simulink model "Simplus_Dual_Automated"  (R2022b)
settings: Solver=ode3  StartTime=0.0  StopTime=35  FixedStep=Ts  RelTol=1e-3  EnableMultiTasking=on
InitFcn:
  | Ts = 100e-6;
model workspace (MAT data in the model file):
  Fbase = 50
  Filter_Ind = 0.00435
  Shunt_C = 2.2e-06
  Test_Interval = 5
  Ts = 0.0001
  VDCref = 48
undefined symbols (not defined in the file): DiscIntNeverNeededParam
libraries: rtpi x45, spsabctodq0Lib x4, spsdq0toabcLib x2, simulink x1
(part 1 of 2)
settings Model: ModifiedByFormat=The MathWorks Inc.  SimulationMode=external  ExtModeTrigDuration=350000  ExtModeLogAll=off  Creator=The MathWorks, Inc.  LastModifiedBy=The MathWorks Inc.
settings SolverCC: AlgebraicLoopSolver=TrustRegion  PositivePriorityOrder=on  AutoInsertRateTranBlk=on
settings DataIOCC: LimitDataPoints=on  SaveFormat=Array  ReturnWorkspaceOutputs=off
settings OptimizationCC: EnhancedBackFolding=on  PassReuseOutputArgsThreshold=0  LocalBlockOutputs=off  EfficientMapNaN2IntZero=off  MaxStackSize=64  OptimizeBlockOrder=speed  DifferentSizesBufferReuse=on
settings DebuggingCC: UnderspecifiedInitializationDetection=Classic  MergeDetectMultiDrivingBlocksExec=none  SolverPrmCheckMsg=warning  ParameterTunabilityLossMsg=error  UnconnectedInputMsg=warning  UnconnectedOutputMsg=warning  UnconnectedLineMsg=warning  AllowSymbolicDim=off  SFUnexpectedBacktrackingDiag=warning  SFNoUnconditionalDefaultTransitionDiag=warning  SFExecutionAtInitializationDiag=none  SFMachineParentedDataDiag=warning  ArithmeticOperatorsInVariantConditions=warning
settings HardwareCC: ProdBitPerPointer=32  ProdBitPerSizeT=32  ProdBitPerPtrDiffT=32  ProdLargestAtomicInteger=Long  ProdLargestAtomicFloat=Double  ProdWordSize=32  ProdHWDeviceType=ARM Compatible->ARM Cortex  UseEmbeddedCoderFeatures=off
settings ModelReferenceCC: EnableRefExpFcnMdlSchedulingChecks=on  PropagateSignalLabelsOutOfModel=off
settings SFSimCC: SimUseLocalCustomCode=off  SimParseCustomCode=off  MATLABDynamicMemAlloc=off  CustomCodeUndefinedFunction=UseInterfaceOnly
settings RTWCC: Description=Simplus  SystemTargetFile=simplus.tlc  TemplateMakefile=simplex.tmf  RTWUseLocalCustomCode=off  RTWUseSimCustomCode=on  Toolchain=Simplus Xenomai ARM32  BuildConfiguration=Faster Runs
settings CodeAppCC: OperatorAnnotations=on  MangleLength=10  StateflowObjectComments=on
settings STFCustomTargetCC: TargetLangStandard=C99 (ISO)  GenerateFullHeader=off  ConcurrentExecutionCompliant=on  GRTInterface=on  UseToolchainInfoCompliant=on  SystemTargetFile=simplus.tlc
settings GRTTargetCC: GenerateFullHeader=off  ParMdlRefBuildCompliant=off  CompOptLevelCompliant=off  CombineOutputUpdateFcns=off  MatFileLogging=off  CPPClassGenCompliant=off  GRTInterface=on  ExtMode=on  ExtModeMexArgs='192.168.10.109', 0, 17725
settings ConfigComp: CovMetricSettings=dw  CovSaveCumulativeToWorkspaceVar=on  CovSaveSingleToWorkspaceVar=on  CovExternalEMLEnable=off  CovSFcnEnable=off

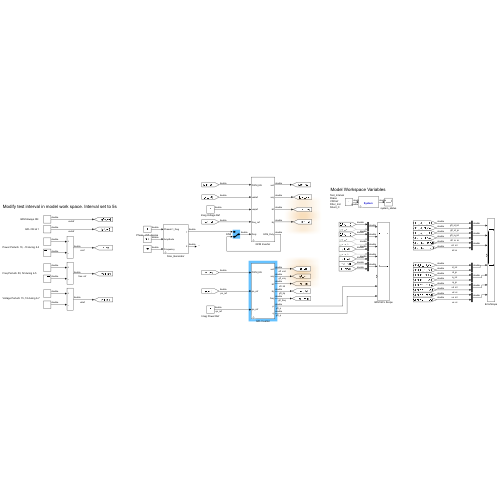
[thumbnail: Simulink's stored preview of the top-level diagram]
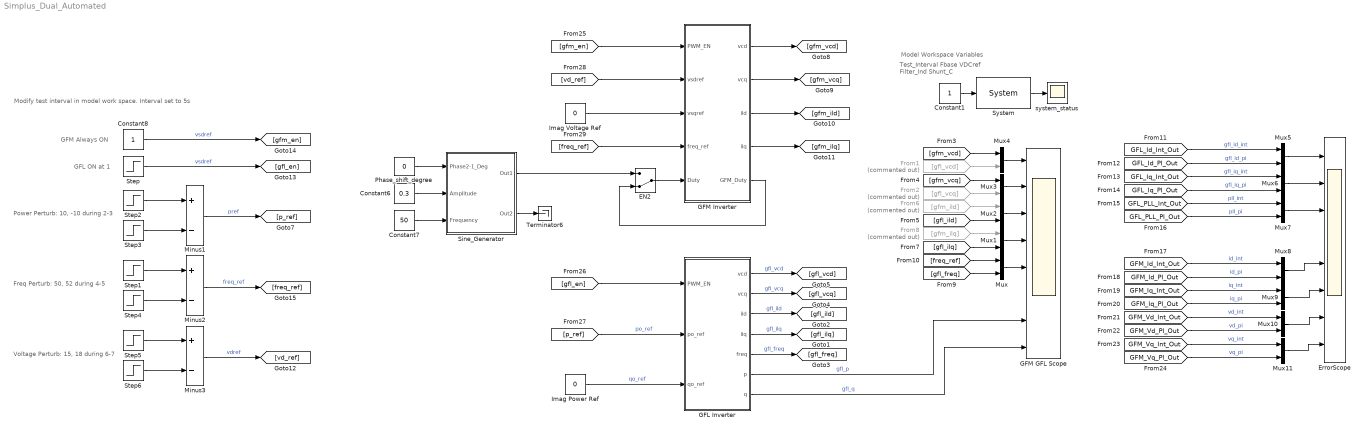
== system Simplus_Dual_Automated ==
  note: Test_Interval
      | Fbase
      | VDCref
      | Filter_Ind
      | Shunt_C
  note: Model Workspace Variables
  note: Modify test interval in model work space. Interval set to 5s
  note: GFM Always ON
  note: Power Perturb: 10, -10 during 2-3
  note: GFL ON at 1
  note: Freq Perturb: 50, 52 during 4-5
  note: Voltage Perturb: 15, 18 during 6-7
  Constant1 : Constant
  Constant6 : Constant  Value=0.3
  Constant7 : Constant  Value=50
  Constant8 : Constant
  EN2 : ManualSwitch  CurrentSetting=0
  ErrorScope : Scope  NumInputPorts=8
  From1 : From  Commented=on  GotoTag=gfl_vcd
      settings: CloseFcn=tagdialog Close
  From2 : From  Commented=on  GotoTag=gfl_vcq
      settings: CloseFcn=tagdialog Close
  From6 : From  Commented=on  GotoTag=gfm_ild
      settings: CloseFcn=tagdialog Close
  From8 : From  Commented=on  GotoTag=gfm_ilq
      settings: CloseFcn=tagdialog Close
  GFL Inverter : Subsystem  mask{Kp_PLL=6.09, Ki_PLL=9.57, IntSat_PLL=10000, Fcutoff=100, Id_Proportional=1.22, Id_Integral=957/16, I_SatLimit=200000}
      mask prompts: Kp_PLL "Proportional (P)"; Ki_PLL "Integral (I)"; IntSat_PLL "Saturator (Offset from 2*pi*Fbase)"; Fcutoff "LPF Cutoff Frequency (Hz)"; Id_Proportional "Proportional (P)"; Id_Integral "Integral (I)"; I_SatLimit "Integrator Saturation"
      mask DialogControl DescGroupVar Prompt: GFL Control Panel
      mask DialogControl DescTextVar Prompt: Modify current controller and PLL gains.
      mask DialogControl ParameterGroupVar_copy Prompt: PLL Parameters
      mask DialogControl Control2 Prompt: LPF is a first order LPF in the form  1/(2pi*f_c s + 1)
      mask DialogControl ParameterGroupVar Prompt: Current Controller Parameters
  GFM GFL Scope : Scope  NumInputPorts=8
  GFM Inverter : Subsystem  mask{Vd_Proportional=0.028, Vd_Integral=8.685*8, V_IntSat=1000, Id_Proportional=0.61, Id_Integral=240/16, I_IntSat=200000}
      mask prompts: Vd_Proportional "Proportional (P)"; Vd_Integral "Integral (I)"; V_IntSat "Integrator Saturator Limit"; Id_Proportional "Proportional (P)"; Id_Integral "Integral (I)"; I_IntSat "Integrator Saturator Limit"
      mask DialogControl DescGroupVar Prompt: GFM Control Panel
      mask DialogControl DescTextVar Prompt: Adjust gains and output/integrator limits for GFM voltage and current controllers
      mask DialogControl ParameterGroupVar_copy Prompt: Voltage Controller
      mask DialogControl ParameterGroupVar Prompt: Current Controller
  Imag Power Ref : Constant  Value=0
  Imag Voltage Ref : Constant  Value=0
  Minus1 : Sum  Inputs=+-
  Minus2 : Sum  Inputs=+-
  Minus3 : Sum  Inputs=+-
  Mux{,1..11} (12 alike) : Mux  Inputs=2
  Phase_shift_degree : Constant  Value=0
  Sine_Generator : Subsystem
  Step : Step  Time=Test_Interval*1
  Step1 : Step  Time=Test_Interval*4  Before=50  After=52
  Step2 : Step  Time=Test_Interval*2  Before=10  After=-10
  Step3 : Step  Time=Test_Interval*3  After=-20
  Step4 : Step  Time=Test_Interval*5  After=2
  Step5 : Step  Time=Test_Interval*6  Before=15  After=18
  Step6 : Step  Time=Test_Interval*7  After=3
  System : rtpi/System  Priority=-100  finger_print=015482637925  sync=Synchronous Series  div=4  estop=NONE
      settings: SourceProductName=Simplus Real-Time
  Terminator6 : Terminator
  system_status : Scope
  wires:
  System/1 -> system_status/1
  Constant1/1 -> System/1
  [gfm_en] -> GFM Inverter/1(PWM_EN)
  [vd_ref] -> GFM Inverter/2(vsdref)
  Imag Voltage Ref/1 -> GFM Inverter/3(vsqref)
  GFM Inverter/1(vcd) -> [gfm_vcd]
  GFM Inverter/2(vcq) -> [gfm_vcq]
  GFM Inverter/3(ild) -> [gfm_ild]
  GFM Inverter/4(ilq) -> [gfm_ilq]
  Mux3/1 -> GFM GFL Scope/2
  Mux4/1 -> GFM GFL Scope/1
  Mux2/1 -> GFM GFL Scope/3
  Mux1/1 -> GFM GFL Scope/4
  Mux/1 -> GFM GFL Scope/5
  [gfl_freq] -> Mux/2
  [freq_ref] -> Mux/1
  [gfl_ilq] -> Mux1/2
  From8/1 -> Mux1/1
  [gfl_ild] -> Mux2/2
  From6/1 -> Mux2/1
  From2/1 -> Mux3/2
  [gfm_vcq] -> Mux3/1
  From1/1 -> Mux4/2
  [gfm_vcd] -> Mux4/1
  Sine_Generator/1(Out1) -> EN2/1
  Constant6/1 -> Sine_Generator/2(Amplitude)
  Constant7/1 -> Sine_Generator/3(Frequency)
  Sine_Generator/2(Out2) -> Terminator6/1
  Phase_shift_degree/1 -> Sine_Generator/1(Phase2-1_Deg)
  GFM Inverter/5(GFM_Duty) -> EN2/2
  EN2/1 -> GFM Inverter/5(Duty)
  [gfl_en] -> GFL Inverter/1(PWM_EN)
  Imag Power Ref/1 -> GFL Inverter/3(qo_ref)  "qo_ref"
  GFL Inverter/2(vcq) -> [gfl_vcq]  "gfl_vcq"
  GFL Inverter/5(freq) -> [gfl_freq]  "gfl_freq"
  [p_ref] -> GFL Inverter/2(po_ref)  "po_ref"
  GFL Inverter/4(ilq) -> [gfl_ilq]  "gfl_ilq"
  GFL Inverter/6(p) -> GFM GFL Scope/7  "gfl_p"
  GFL Inverter/3(ild) -> [gfl_ild]  "gfl_ild"
  GFL Inverter/1(vcd) -> [gfl_vcd]  "gfl_vcd"
  GFL Inverter/7(q) -> GFM GFL Scope/8  "gfl_q"
  [GFL_Id_PI_Out] -> Mux5/2  "gfl_id_pi"
  Mux5/1 -> ErrorScope/1
  [GFL_Id_Int_Out] -> Mux5/1  "gfl_id_int"
  [GFL_Iq_Int_Out] -> Mux6/1  "gfl_iq_int"
  [GFL_Iq_PI_Out] -> Mux6/2  "gfl_iq_pi"
  Mux6/1 -> ErrorScope/2
  [GFL_PLL_Int_Out] -> Mux7/1  "pll_int"
  Mux7/1 -> ErrorScope/3
  [GFL_PLL_PI_Out] -> Mux7/2  "pll_pi"
  [GFM_Id_Int_Out] -> Mux8/1  "id_int"
  [GFM_Id_PI_Out] -> Mux8/2  "id_pi"
  Mux10/1 -> ErrorScope/7
  Mux8/1 -> ErrorScope/5
  [GFM_Vd_Int_Out] -> Mux10/1  "vd_int"
  [GFM_Iq_Int_Out] -> Mux9/1  "iq_int"
  Mux9/1 -> ErrorScope/6
  [GFM_Iq_PI_Out] -> Mux9/2  "iq_pi"
  [GFM_Vd_PI_Out] -> Mux10/2  "vd_pi"
  Mux11/1 -> ErrorScope/8
  [GFM_Vq_Int_Out] -> Mux11/1  "vq_int"
  [GFM_Vq_PI_Out] -> Mux11/2  "vq_pi"
  Step2/1 -> Minus1/1
  Step3/1 -> Minus1/2
  Step/1 -> [gfl_en]  "vsdref"
  Minus1/1 -> [p_ref]  "pref"
  Constant8/1 -> [gfm_en]  "vsdref"
  Minus2/1 -> [freq_ref]  "freq_ref"
  Step4/1 -> Minus2/2
  Step1/1 -> Minus2/1
  [freq_ref] -> GFM Inverter/4(freq_ref)
  Minus3/1 -> [vd_ref]  "vdref"
  Step6/1 -> Minus3/2
  Step5/1 -> Minus3/1

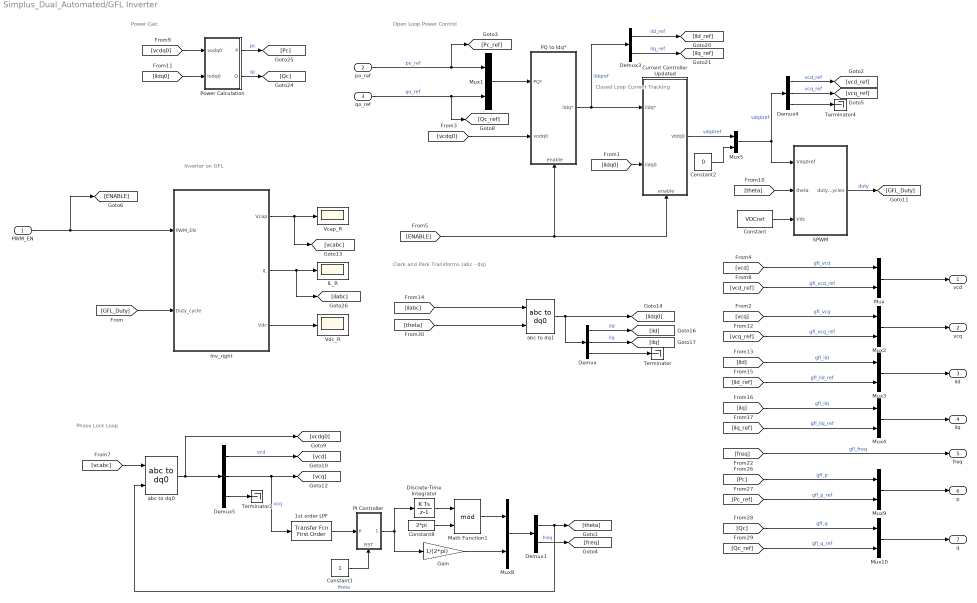
== system Simplus_Dual_Automated/GFL Inverter ==
  note: Clark and Park Transforms (abc - dq)
  note: Closed Loop Current Tracking
  note: Phase Lock Loop
  note: Inverter on GFL
  note: Power Calc
  note: Open Loop Power Control
  PWM_EN : Inport
  po_ref : Inport  Port=2
  qo_ref : Inport  Port=3
  1st order LPF : simulink/Discrete/Transfer Fcn First Order  PoleZ=exp(-2*pi*Fcutoff*Ts)  ICPrevOutput=0.0  DoSatur=off
  Constant : Constant  Value=VDCref
  Constant1 : Constant
  Constant2 : Constant  Value=0
  Constant8 : Constant  Value=2*pi
  Current Controller Updated : Subsystem
      settings: PortSchema="{\"entries\":[{\"content\":{\"sides\":[{\"content\":{\"connectorIds\":[\"In1\",\"In2\"]},\"type\":\"ConnectorPlacement.EquallySpacedRectSide\",\"uuid\":\"134caf41-c34b-48d0-a71a-522329c40d8c\"},{\"content\":{\"connectorIds\":[\"Out1\"],\"side\":\"RIGHT\"},\"type\":\"ConnectorPlacement.EquallySpacedRectSide\",\"uuid\":\"de6d8359-09d9-4cb7-8990-bc4b6d48f18d\"},{\"content\":{\"connectorIds\":[],\"side\":\"TOP\"},\"type\":\"ConnectorPlacement.EquallySpacedRectSide\",\"uuid\":\"e2785d07-2ead-4d42-94ac-8025f550e46a\"},{\"content\":{\"connectorIds\":[\"In3\"],\"side\":\"BOTTOM\"},\"type\":\"ConnectorPlacement.EquallySpacedRectSide\",\"uuid\":\"a912a274-012c-4cba-911c-beb79bb7dc91\"}]},\"type\":\"ConnectorPlacement.EquallySpacedConnector\",\"uuid\":\"3c498838-bb9a-4b09-bf48-00f71cabf7b4\"}],\"packageUris\":[\"http://schema.mathworks.com/mf0/Connector/R2020b\"],\"version\":\"1.0\"}"
  Demux : Demux  Outputs=3
  Demux1 : Demux  Outputs=2
  Demux3 : Demux  Outputs=2
  Demux4 : Demux  Outputs=3
  Demux5 : Demux  Outputs=3
  Discrete-Time Integrator : DiscreteIntegrator  SampleTime=Ts  ICPrevOutput=DiscIntNeverNeededParam  ICPrevScaledInput=DiscIntNeverNeededParam
  Gain : Gain  Gain=1/(2*pi)
  IL_R : Scope
  Inv_right : Subsystem
  Math Function1 : Math  Operator=mod  SignedPower=on
  Mux{,1..5,8..10} (9 alike) : Mux  Inputs=2
  PI Controller : Subsystem
      settings: PortSchema="{\"entries\":[{\"content\":{\"sides\":[{\"content\":{\"connectorIds\":[\"In1\"]},\"type\":\"ConnectorPlacement.EquallySpacedRectSide\",\"uuid\":\"de74edf3-48e0-492f-8bd8-cb8fa34f4920\"},{\"content\":{\"connectorIds\":[\"Out1\"],\"side\":\"RIGHT\"},\"type\":\"ConnectorPlacement.EquallySpacedRectSide\",\"uuid\":\"732ba37e-c2f5-4a41-96c7-cf5d66f1810a\"},{\"content\":{\"connectorIds\":[],\"side\":\"TOP\"},\"type\":\"ConnectorPlacement.EquallySpacedRectSide\",\"uuid\":\"cc9767f0-3de2-493b-9176-a3d2c83c4b10\"},{\"content\":{\"connectorIds\":[\"In2\"],\"side\":\"BOTTOM\"},\"type\":\"ConnectorPlacement.EquallySpacedRectSide\",\"uuid\":\"a440190f-f792-4428-a915-fb5e20f94e16\"}]},\"type\":\"ConnectorPlacement.EquallySpacedConnector\",\"uuid\":\"ab91a7bc-5a4b-4de4-8ccc-ccc371bac732\"}],\"packageUris\":[\"http://schema.mathworks.com/mf0/Connector/R2020b\"],\"version\":\"1.0\"}"
  PQ to Idq* : Subsystem
      settings: PortSchema="{\"entries\":[{\"content\":{\"sides\":[{\"content\":{\"connectorIds\":[\"In1\",\"In2\"]},\"type\":\"ConnectorPlacement.EquallySpacedRectSide\",\"uuid\":\"5271b3ed-46a4-4113-9b69-458d23b85fa2\"},{\"content\":{\"connectorIds\":[\"Out1\"],\"side\":\"RIGHT\"},\"type\":\"ConnectorPlacement.EquallySpacedRectSide\",\"uuid\":\"00fb532b-4b50-4607-a5c4-cd74a5a5fc42\"},{\"content\":{\"connectorIds\":[],\"side\":\"TOP\"},\"type\":\"ConnectorPlacement.EquallySpacedRectSide\",\"uuid\":\"05671b8e-b1fa-45d3-a4a8-1640aa1af326\"},{\"content\":{\"connectorIds\":[\"In3\"],\"side\":\"BOTTOM\"},\"type\":\"ConnectorPlacement.EquallySpacedRectSide\",\"uuid\":\"cfa1ca65-6f63-4245-906b-c8bf76b96ed3\"}]},\"type\":\"ConnectorPlacement.EquallySpacedConnector\",\"uuid\":\"bf062c94-390f-4409-83d1-f8a32d59f496\"}],\"packageUris\":[\"http://schema.mathworks.com/mf0/Connector/R2020b\"],\"version\":\"1.0\"}"
  Power Calculation : Subsystem
  SPWM : Subsystem
  Terminator : Terminator
  Terminator2 : Terminator
  Terminator4 : Terminator
  Vcap_R : Scope
  Vdc_R : Scope
  abc to dq0 : spsabctodq0Lib/abc to dq0  Alignment=90 degrees behind phase A axis
  abc to dq1 : spsabctodq0Lib/abc to dq0  Alignment=90 degrees behind phase A axis
  vcd : Outport
  vcq : Outport  Port=2
  ild : Outport  Port=3
  ilq : Outport  Port=4
  freq : Outport  Port=5
  p : Outport  Port=6
  q : Outport  Port=7
  wires:
  [ild] -> Mux3/1  "gfl_ild"
  Demux1/1 -> abc to dq0/2, [theta]  "theta"
  Inv_right/2(IL) -> [ilabc], IL_R/1
  Inv_right/1(Vcap) -> [vcabc], Vcap_R/1
  Mux5/1 -> Demux4/1, SPWM/1(Vdq0ref)  "vdq0ref"
  Demux3/1 -> [ild_ref]  "ild_ref"
  Demux5/2 -> 1st order LPF/1, [vcq]  "vcq"
  Math Function1/1 -> Mux8/1
  [ild_ref] -> Mux3/2  "gfl_ild_ref"
  Power Calculation/1(P) -> [Pc]  "pc"
  [Pc_ref] -> Mux9/2  "gfl_p_ref"
  Power Calculation/2(Q) -> [Qc]  "qc"
  [vcabc] -> abc to dq0/1
  Constant/1 -> SPWM/3(Vdc)
  Demux/2 -> [ilq]  "ilq"
  Demux3/2 -> [ilq_ref]  "ilq_ref"
  [theta] -> SPWM/2(theta)
  Demux/3 -> Terminator/1
  [Qc] -> Mux10/1  "gfl_q"
  SPWM/1(duty_cycles) -> [GFL_Duty]  "duty"
  abc to dq0/1 -> [vcdq0], Demux5/1
  qo_ref/1 -> [Qc_ref], Mux1/2  "qo_ref"
  Demux4/2 -> [vcq_ref]  "vcq_ref"
  [ilq_ref] -> Mux4/2  "gfl_ilq_ref"
  Demux/1 -> [ild]  "ild"
  PQ to Idq*/1(iIdq*) -> Current Controller Updated/1(ildq*), Demux3/1  "ildqref"
  Demux4/3 -> Terminator4/1
  [vcq_ref] -> Mux2/2  "gfl_vcq_ref"
  [vcdq0] -> Power Calculation/1(vodq0)
  Discrete-Time Integrator/1 -> Math Function1/1
  PWM_EN/1 -> Inv_right/1(PWM_EN), [ENABLE]
  [theta] -> abc to dq1/2
  Gain/1 -> Mux8/2
  [vcd] -> Mux/1  "gfl_vcd"
  Mux1/1 -> PQ to Idq*/1(PQ*)
  Constant8/1 -> Math Function1/2
  [vcd_ref] -> Mux/2  "gfl_vcd_ref"
  Demux1/2 -> [freq]  "freq"
  [vcq] -> Mux2/1  "gfl_vcq"
  abc to dq1/1 -> [ildq0], Demux/1
  [ilq] -> Mux4/1  "gfl_ilq"
  Mux8/1 -> Demux1/1
  [ildq0] -> Current Controller Updated/2(ildq0)
  [Pc] -> Mux9/1  "gfl_p"
  Demux5/1 -> [vcd]  "vcd"
  [vcdq0] -> PQ to Idq*/2(vodq0)
  Demux5/3 -> Terminator2/1
  Inv_right/3(Vdc) -> Vdc_R/1
  [ildq0] -> Power Calculation/2(iodq0)
  [Qc_ref] -> Mux10/2  "gfl_q_ref"
  [ilabc] -> abc to dq1/1
  [GFL_Duty] -> Inv_right/2(Duty_cycle)
  po_ref/1 -> [Pc_ref], Mux1/1  "po_ref"
  Demux4/1 -> [vcd_ref]  "vcd_ref"
  PI Controller/1(Out) -> Gain/1, Discrete-Time Integrator/1
  Mux4/1 -> ilq/1
  Mux/1 -> vcd/1
  Mux3/1 -> ild/1
  Mux9/1 -> p/1
  Mux10/1 -> q/1
  Mux2/1 -> vcq/1
  [freq] -> freq/1  "gfl_freq"
  [ENABLE] -> Current Controller Updated/3(enable), PQ to Idq*/3(enable)
  Current Controller Updated/1(vtdq0) -> Mux5/1  "vdq0ref"
  Constant2/1 -> Mux5/2
  1st order LPF/1 -> PI Controller/1(e)
  Constant1/1 -> PI Controller/2(RST)

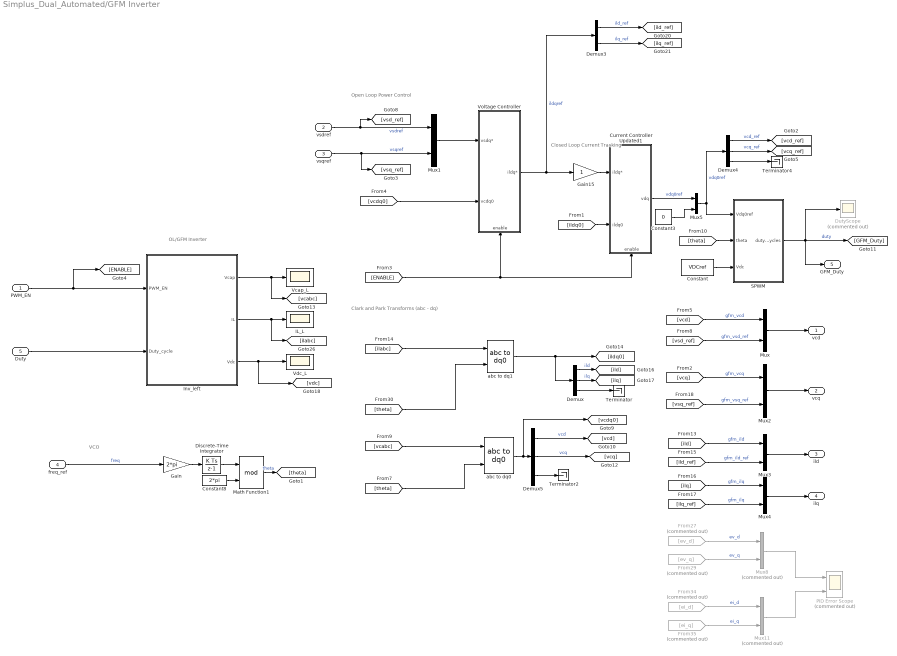
== system Simplus_Dual_Automated/GFM Inverter ==
  note: OL/GFM Inverter
  note: Open Loop Power Control
  note: VCO
  note: Clark and Park Transforms (abc - dq)
  note: Closed Loop Current Tracking
  PWM_EN : Inport
  vsdref : Inport  Port=2
  vsqref : Inport  Port=3
  freq_ref : Inport  Port=4
  Duty : Inport  Port=5
  Constant : Constant  Value=VDCref
  Constant3 : Constant  Value=0
  Constant8 : Constant  Value=2*pi
  Current Controller Updated1 : Subsystem
      settings: PortSchema="{\"entries\":[{\"content\":{\"sides\":[{\"content\":{\"connectorIds\":[\"In1\",\"In2\"]},\"type\":\"ConnectorPlacement.EquallySpacedRectSide\",\"uuid\":\"134caf41-c34b-48d0-a71a-522329c40d8c\"},{\"content\":{\"connectorIds\":[\"Out1\"],\"side\":\"RIGHT\"},\"type\":\"ConnectorPlacement.EquallySpacedRectSide\",\"uuid\":\"de6d8359-09d9-4cb7-8990-bc4b6d48f18d\"},{\"content\":{\"connectorIds\":[],\"side\":\"TOP\"},\"type\":\"ConnectorPlacement.EquallySpacedRectSide\",\"uuid\":\"e2785d07-2ead-4d42-94ac-8025f550e46a\"},{\"content\":{\"connectorIds\":[\"In3\"],\"side\":\"BOTTOM\"},\"type\":\"ConnectorPlacement.EquallySpacedRectSide\",\"uuid\":\"a912a274-012c-4cba-911c-beb79bb7dc91\"}]},\"type\":\"ConnectorPlacement.EquallySpacedConnector\",\"uuid\":\"3c498838-bb9a-4b09-bf48-00f71cabf7b4\"}],\"packageUris\":[\"http://schema.mathworks.com/mf0/Connector/R2020b\"],\"version\":\"1.0\"}"
  Demux : Demux  Outputs=3
  Demux3 : Demux  Outputs=2
  Demux4 : Demux  Outputs=3
  Demux5 : Demux  Outputs=3
  Discrete-Time Integrator : DiscreteIntegrator  SampleTime=Ts  ICPrevOutput=DiscIntNeverNeededParam  ICPrevScaledInput=DiscIntNeverNeededParam
  DutyScope : Scope  Commented=on
  From27 : From  Commented=on  GotoTag=ev_d
      settings: CloseFcn=tagdialog Close
  From29 : From  Commented=on  GotoTag=ev_q
      settings: CloseFcn=tagdialog Close
  From34 : From  Commented=on  GotoTag=ei_d
      settings: CloseFcn=tagdialog Close
  From35 : From  Commented=on  GotoTag=ei_q
      settings: CloseFcn=tagdialog Close
  Gain : Gain  Gain=2*pi
  Gain15 : Gain
  IL_L : Scope
  Inv_left : Subsystem
  Math Function1 : Math  Operator=mod  SignedPower=on
  Mux{,1..5} (6 alike) : Mux  Inputs=2
  Mux11 : Mux  Commented=on  Inputs=2
  Mux8 : Mux  Commented=on  Inputs=2
  PID Error Scope : Scope  Commented=on  NumInputPorts=2
  SPWM : Subsystem
  Terminator : Terminator
  Terminator2 : Terminator
  Terminator4 : Terminator
  Vcap_L : Scope
  Vdc_L : Scope
  Voltage Controller : Subsystem
      settings: PortSchema="{\"entries\":[{\"content\":{\"sides\":[{\"content\":{\"connectorIds\":[\"In1\",\"In2\"]},\"type\":\"ConnectorPlacement.EquallySpacedRectSide\",\"uuid\":\"134caf41-c34b-48d0-a71a-522329c40d8c\"},{\"content\":{\"connectorIds\":[\"Out1\"],\"side\":\"RIGHT\"},\"type\":\"ConnectorPlacement.EquallySpacedRectSide\",\"uuid\":\"de6d8359-09d9-4cb7-8990-bc4b6d48f18d\"},{\"content\":{\"connectorIds\":[],\"side\":\"TOP\"},\"type\":\"ConnectorPlacement.EquallySpacedRectSide\",\"uuid\":\"e2785d07-2ead-4d42-94ac-8025f550e46a\"},{\"content\":{\"connectorIds\":[\"In3\"],\"side\":\"BOTTOM\"},\"type\":\"ConnectorPlacement.EquallySpacedRectSide\",\"uuid\":\"a912a274-012c-4cba-911c-beb79bb7dc91\"}]},\"type\":\"ConnectorPlacement.EquallySpacedConnector\",\"uuid\":\"3c498838-bb9a-4b09-bf48-00f71cabf7b4\"}],\"packageUris\":[\"http://schema.mathworks.com/mf0/Connector/R2020b\"],\"version\":\"1.0\"}"
  abc to dq0 : spsabctodq0Lib/abc to dq0  Alignment=90 degrees behind phase A axis
  abc to dq1 : spsabctodq0Lib/abc to dq0  Alignment=90 degrees behind phase A axis
  vcd : Outport
  vcq : Outport  Port=2
  ild : Outport  Port=3
  ilq : Outport  Port=4
  GFM_Duty : Outport  Port=5
  wires:
  Inv_left/3(Vdc) -> Vdc_L/1, [vdc]
  [theta] -> SPWM/2(theta)
  vsdref/1 -> [vsd_ref], Mux1/1  "vsdref"
  Inv_left/1(Vcap) -> Vcap_L/1, [vcabc]
  Demux3/2 -> [ilq_ref]  "ilq_ref"
  Constant8/1 -> Math Function1/2
  Inv_left/2(IL) -> IL_L/1, [ilabc]
  Mux5/1 -> Demux4/1, SPWM/1(Vdq0ref)  "vdq0ref"
  Demux5/2 -> [vcq]  "vcq"
  [vcd] -> Mux/1  "gfm_vcd"
  Gain15/1 -> Current Controller Updated1/1(ildq*)
  Demux5/1 -> [vcd]  "vcd"
  [ild] -> Mux3/1  "gfm_ild"
  Mux/1 -> vcd/1
  PWM_EN/1 -> Inv_left/1(PWM_EN), [ENABLE]
  Demux/2 -> [ilq]  "ilq"
  Demux5/3 -> Terminator2/1
  [ENABLE] -> Voltage Controller/3(enable), Current Controller Updated1/3(enable)
  Gain/1 -> Discrete-Time Integrator/1
  Mux1/1 -> Voltage Controller/1(vsdq*)
  [theta] -> abc to dq0/2
  [ild_ref] -> Mux3/2  "gfm_ild_ref"
  Demux/3 -> Terminator/1
  [ilq] -> Mux4/1  "gfm_ilq"
  [ilabc] -> abc to dq1/1
  abc to dq1/1 -> [ildq0], Demux/1
  [ildq0] -> Current Controller Updated1/2(ildq0)
  [vsq_ref] -> Mux2/2  "gfm_vsq_ref"
  [vcq] -> Mux2/1  "gfm_vcq"
  [vsd_ref] -> Mux/2  "gfm_vsd_ref"
  Demux4/2 -> [vcq_ref]  "vcq_ref"
  Voltage Controller/1(ildq*) -> Demux3/1, Gain15/1  "ildqref"
  [ilq_ref] -> Mux4/2  "gfm_ilq"
  Demux/1 -> [ild]  "ild"
  [theta] -> abc to dq1/2
  SPWM/1(duty_cycles) -> GFM_Duty/1, DutyScope/1, [GFM_Duty]  "duty"
  freq_ref/1 -> Gain/1  "freq"
  abc to dq0/1 -> [vcdq0], Demux5/1
  Constant/1 -> SPWM/3(Vdc)
  Math Function1/1 -> [theta]  "theta"
  Demux3/1 -> [ild_ref]  "ild_ref"
  Mux3/1 -> ild/1
  vsqref/1 -> [vsq_ref], Mux1/2  "vsqref"
  Discrete-Time Integrator/1 -> Math Function1/1
  Demux4/3 -> Terminator4/1
  Demux4/1 -> [vcd_ref]  "vcd_ref"
  [vcabc] -> abc to dq0/1
  Mux2/1 -> vcq/1
  Mux4/1 -> ilq/1
  From34/1 -> Mux11/1  "ei_d"
  Mux11/1 -> PID Error Scope/2
  From27/1 -> Mux8/1  "ev_d"
  Mux8/1 -> PID Error Scope/1
  From29/1 -> Mux8/2  "ev_q"
  From35/1 -> Mux11/2  "ei_q"
  [vcdq0] -> Voltage Controller/2(vcdq0)
  Duty/1 -> Inv_left/2(Duty_cycle)
  Current Controller Updated1/1(vdq) -> Mux5/1  "vdq0ref"
  Constant3/1 -> Mux5/2

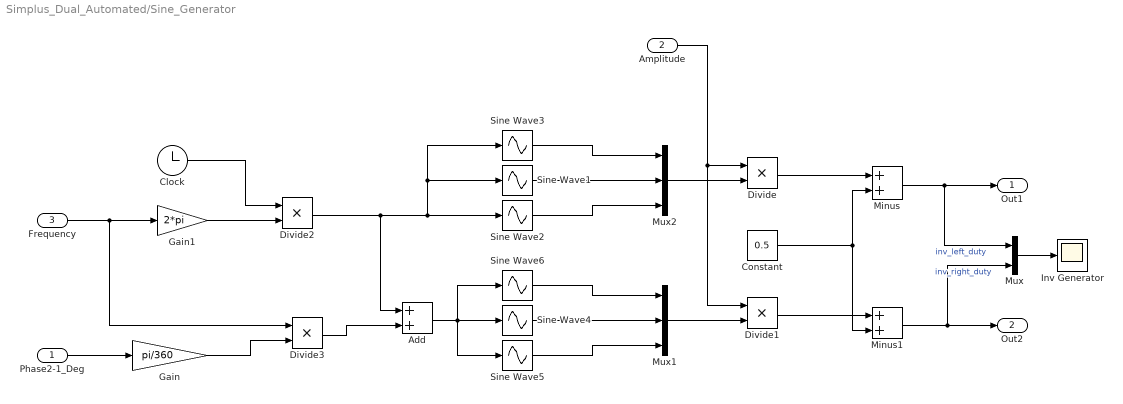
== system Simplus_Dual_Automated/Sine_Generator ==
  Phase2-1_Deg : Inport
  Amplitude : Inport  Port=2
  Frequency : Inport  Port=3
  Add : Sum
  Clock : Clock
  Constant : Constant  Value=0.5
  Divide{,1..3} (4 alike) : Product  Inputs=**
  Gain : Gain  Gain=pi/360
  Gain1 : Gain  Gain=2*pi
  Inv Generator : Scope
  Minus : Sum
  Minus1 : Sum
  Mux : Mux  Inputs=2
  Mux1 : Mux  Inputs=3
  Mux2 : Mux  Inputs=3
  Sine Wave1 : Sin  TimeSource=Use external signal  Phase=-2*pi/3
  Sine Wave2 : Sin  TimeSource=Use external signal  Phase=2*pi/3
  Sine Wave3 : Sin  TimeSource=Use external signal
  Sine Wave4 : Sin  TimeSource=Use external signal  Phase=-2*pi/3
  Sine Wave5 : Sin  TimeSource=Use external signal  Phase=2*pi/3
  Sine Wave6 : Sin  TimeSource=Use external signal
  Out1 : Outport
  Out2 : Outport  Port=2
  wires:
  Add/1 -> Sine Wave6/1, Sine Wave5/1, Sine Wave4/1
  Sine Wave3/1 -> Mux2/1
  Divide2/1 -> Add/1, Sine Wave1/1, Sine Wave3/1, Sine Wave2/1
  Sine Wave6/1 -> Mux1/1
  Divide3/1 -> Add/2
  Sine Wave5/1 -> Mux1/3
  Sine Wave4/1 -> Mux1/2
  Sine Wave1/1 -> Mux2/2
  Sine Wave2/1 -> Mux2/3
  Minus/1 -> Out1/1, Mux/1  "inv_left_duty"
  Phase2-1_Deg/1 -> Gain/1
  Mux2/1 -> Divide/2
  Mux1/1 -> Divide1/2
  Amplitude/1 -> Divide/1, Divide1/1
  Gain1/1 -> Divide2/2
  Frequency/1 -> Divide3/1, Gain1/1
  Divide/1 -> Minus/1
  Divide1/1 -> Minus1/1
  Constant/1 -> Minus1/2, Minus/2
  Clock/1 -> Divide2/1
  Gain/1 -> Divide3/2
  Minus1/1 -> Out2/1, Mux/2  "inv_right_duty"
  Mux/1 -> Inv Generator/1

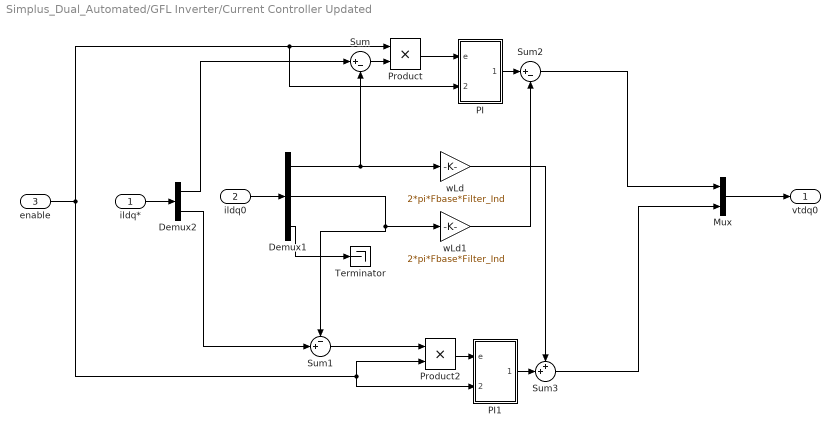
== system Simplus_Dual_Automated/GFL Inverter/Current Controller Updated ==
  ildq* : Inport
  ildq0 : Inport  Port=2
  enable : Inport  Port=3
  Demux1 : Demux  Outputs=3
  Demux2 : Demux  Outputs=2
  Mux : Mux  Inputs=2
  PI : Subsystem
  PI1 : Subsystem
  Product : Product  RndMeth=Zero
  Product2 : Product  RndMeth=Zero
  Sum : Sum  Inputs=|+-
  Sum1 : Sum  Inputs=-+|
  Sum2 : Sum  Inputs=|+-
  Sum3 : Sum  Inputs=++|
  Terminator : Terminator
  wLd : Gain  Gain=2*pi*Fbase*Filter_Ind
  wLd1 : Gain  Gain=2*pi*Fbase*Filter_Ind
  vtdq0 : Outport
  wires:
  Sum2/1 -> Mux/1
  Sum3/1 -> Mux/2
  ildq0/1 -> Demux1/1
  Mux/1 -> vtdq0/1
  Demux1/3 -> Terminator/1
  ildq*/1 -> Demux2/1
  Demux2/1 -> Sum/1
  Demux2/2 -> Sum1/2
  Product/1 -> PI/1(e)
  Sum1/1 -> Product2/1
  PI/1(Out) -> Sum2/1
  wLd/1 -> Sum3/1
  wLd1/1 -> Sum2/2
  PI1/1(Out) -> Sum3/2
  Demux1/2 -> Sum1/1, wLd1/1
  Demux1/1 -> wLd/1, Sum/2
  Product2/1 -> PI1/1(e)
  Sum/1 -> Product/2
  enable/1 -> Product/1, PI/2(RST), PI1/2(RST), Product2/2

== system Simplus_Dual_Automated/GFL Inverter/Inv_right ==
  PWM_EN : Inport
  Duty_cycle : Inport  Port=2
  Switches : Subsystem
  measurement : Subsystem
  Vcap : Outport
  IL : Outport  Port=2
  Vdc : Outport  Port=3
  wires:
  measurement/1(Vcap) -> Vcap/1
  measurement/2(IL) -> IL/1
  measurement/3(Vdc) -> Vdc/1
  PWM_EN/1 -> Switches/1(PWM_EN)
  Duty_cycle/1 -> Switches/2(Duty_cycle)

== system Simplus_Dual_Automated/GFL Inverter/PI Controller ==
  e : Inport
  RST : Inport  Port=2
  Discrete-Time Integrator : DiscreteIntegrator  gainval=1  ExternalReset=either  InitialCondition=2*pi*Fbase  SampleTime=Ts  LimitOutput=on  UpperSaturationLimit=2*pi*Fbase + IntSat_PLL  LowerSaturationLimit=2*pi*Fbase - IntSat_PLL  ICPrevOutput=DiscIntNeverNeededParam  ICPrevScaledInput=DiscIntNeverNeededParam
  Ki : Gain  Gain=Ki_PLL  SaturateOnIntegerOverflow=on  OutDataTypeStr=Inherit: Same as input  ParamDataTypeStr=Inherit: Same as input
  Kp : Gain  Gain=Kp_PLL  SaturateOnIntegerOverflow=on  OutDataTypeStr=Inherit: Same as input  ParamDataTypeStr=Inherit: Same as input
  Sum4 : Sum  SaturateOnIntegerOverflow=on
  Out : Outport
  tag scope: GFL_PLL_Int_Out=global, GFL_PLL_PI_Out=global
  wires:
  Ki/1 -> Discrete-Time Integrator/1
  Kp/1 -> Sum4/1
  e/1 -> Ki/1, Kp/1
  RST/1 -> Discrete-Time Integrator/2
  Discrete-Time Integrator/1 -> [GFL_PLL_Int_Out], Sum4/2
  Sum4/1 -> [GFL_PLL_PI_Out], Out/1

== system Simplus_Dual_Automated/GFL Inverter/PQ to Idq* ==
  note: PQ Calculation
  PQ* : Inport
  vodq0 : Inport  Port=2
  enable : Inport  Port=3
  Mux1 : Mux  Inputs=2
  Mux4 : Mux  Inputs=2
  P->Id : Fcn  Expr=(u[1]*u[3]+u[2]*u[4])/(u[3]*u[3]+u[4]*u[4])
  Product : Product  RndMeth=Zero
  Q->Iq : Fcn  Expr=-(-u[1]*u[4]+u[2]*u[3])/(u[3]*u[3]+u[4]*u[4])
  iIdq* : Outport
  wires:
  enable/1 -> Product/2
  Product/1 -> Mux1/1
  Mux1/1 -> P->Id/1, Q->Iq/1
  P->Id/1 -> Mux4/1
  Q->Iq/1 -> Mux4/2
  Mux4/1 -> iIdq*/1
  vodq0/1 -> Mux1/2
  PQ*/1 -> Product/1

== system Simplus_Dual_Automated/GFL Inverter/Power Calculation ==
  vodq0 : Inport
  iodq0 : Inport  Port=2
  Demux2 : Demux  Outputs=3
  Demux3 : Demux  Outputs=3
  Filter p : DiscreteTransferFcn  Numerator=250*2*pi*Ts  Denominator=[1 ((250*2*pi*Ts)-1)]  SampleTime=Ts
  Filter q : DiscreteTransferFcn  Numerator=250*2*pi*Ts  Denominator=[1 ((250*2*pi*Ts)-1)]  SampleTime=Ts
  Power calculator : Subsystem
  Terminator : Terminator
  Terminator1 : Terminator
  P : Outport
  Q : Outport  Port=2
  wires:
  vodq0/1 -> Demux2/1
  Demux2/1 -> Power calculator/1(Vd)
  Demux2/2 -> Power calculator/2(Vq)
  Demux3/1 -> Power calculator/3(Id)
  Demux3/2 -> Power calculator/4(Iq)
  iodq0/1 -> Demux3/1
  Power calculator/1(p) -> Filter p/1  "P"
  Power calculator/2(q) -> Filter q/1  "Q"
  Demux2/3 -> Terminator/1
  Demux3/3 -> Terminator1/1
  Filter p/1 -> P/1
  Filter q/1 -> Q/1

== system Simplus_Dual_Automated/GFL Inverter/SPWM ==
  Vdq0ref : Inport
  theta : Inport  Port=2
  Vdc : Inport  Port=3
  Constant : Constant
  Divide : Product  Inputs=*/
  Gain : Gain  Gain=1/2
  Gain13 : Gain  Gain=2
  Plus : Sum
  Saturation : Saturate  UpperLimit=0.9  LowerLimit=0.1
  dq0 to abc : spsdq0toabcLib/dq0 to abc  Alignment=90 degrees behind phase A axis
  duty_cycles : Outport
  wires:
  Vdq0ref/1 -> dq0 to abc/1
  Gain/1 -> Saturation/1
  theta/1 -> dq0 to abc/2
  Constant/1 -> Plus/2
  Plus/1 -> Gain/1
  Saturation/1 -> duty_cycles/1
  dq0 to abc/1 -> Gain13/1
  Gain13/1 -> Divide/1
  Vdc/1 -> Divide/2
  Divide/1 -> Plus/1

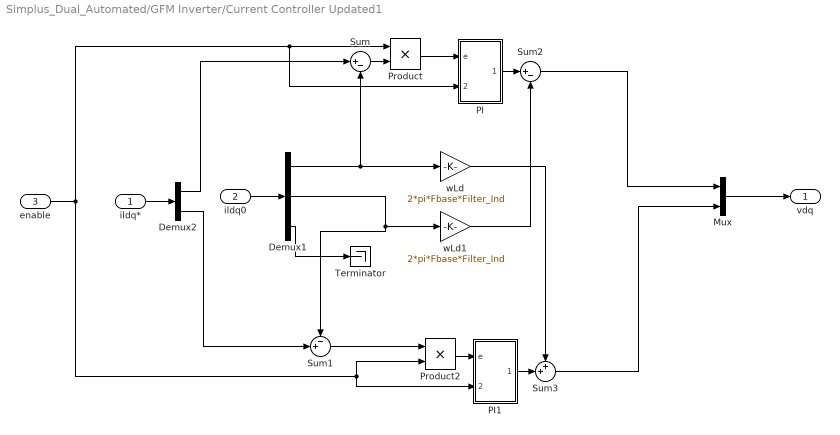
== system Simplus_Dual_Automated/GFM Inverter/Current Controller Updated1 ==
  ildq* : Inport
  ildq0 : Inport  Port=2
  enable : Inport  Port=3
  Demux1 : Demux  Outputs=3
  Demux2 : Demux  Outputs=2
  Mux : Mux  Inputs=2
  PI : Subsystem
  PI1 : Subsystem
  Product : Product  RndMeth=Zero
  Product2 : Product  RndMeth=Zero
  Sum : Sum  Inputs=|+-
  Sum1 : Sum  Inputs=-+|
  Sum2 : Sum  Inputs=|+-
  Sum3 : Sum  Inputs=++|
  Terminator : Terminator
  wLd : Gain  Gain=2*pi*Fbase*Filter_Ind
  wLd1 : Gain  Gain=2*pi*Fbase*Filter_Ind
  vdq : Outport
  wires:
  Sum2/1 -> Mux/1
  Sum3/1 -> Mux/2
  ildq0/1 -> Demux1/1
  Mux/1 -> vdq/1
  Demux1/3 -> Terminator/1
  ildq*/1 -> Demux2/1
  Demux2/1 -> Sum/1
  Demux2/2 -> Sum1/2
  Product/1 -> PI/1(e)
  Sum1/1 -> Product2/1
  PI/1(Out) -> Sum2/1
  wLd/1 -> Sum3/1
  wLd1/1 -> Sum2/2
  PI1/1(Out) -> Sum3/2
  Demux1/2 -> Sum1/1, wLd1/1
  Demux1/1 -> wLd/1, Sum/2
  Product2/1 -> PI1/1(e)
  Sum/1 -> Product/2
  enable/1 -> Product/1, PI/2(RST), PI1/2(RST), Product2/2

== system Simplus_Dual_Automated/GFM Inverter/Inv_left ==
  PWM_EN : Inport
  Duty_cycle : Inport  Port=2
  Switches : Subsystem
  measurement : Subsystem
  Vcap : Outport
  IL : Outport  Port=2
  Vdc : Outport  Port=3
  wires:
  Duty_cycle/1 -> Switches/2(Duty_cycle)
  PWM_EN/1 -> Switches/1(PWM_EN)
  measurement/3(Vdc) -> Vdc/1
  measurement/2(IL) -> IL/1
  measurement/1(Vcap) -> Vcap/1

== system Simplus_Dual_Automated/GFM Inverter/SPWM ==
  Vdq0ref : Inport
  theta : Inport  Port=2
  Vdc : Inport  Port=3
  Constant : Constant
  Divide : Product  Inputs=*/
  Gain : Gain  Gain=1/2
  Gain13 : Gain  Gain=2
  Plus : Sum
  Saturation : Saturate  UpperLimit=0.9  LowerLimit=0.1
  dq0 to abc : spsdq0toabcLib/dq0 to abc  Alignment=90 degrees behind phase A axis
  duty_cycles : Outport
  wires:
  Vdq0ref/1 -> dq0 to abc/1
  Gain/1 -> Saturation/1
  theta/1 -> dq0 to abc/2
  Constant/1 -> Plus/2
  Plus/1 -> Gain/1
  Saturation/1 -> duty_cycles/1
  dq0 to abc/1 -> Gain13/1
  Gain13/1 -> Divide/1
  Vdc/1 -> Divide/2
  Divide/1 -> Plus/1

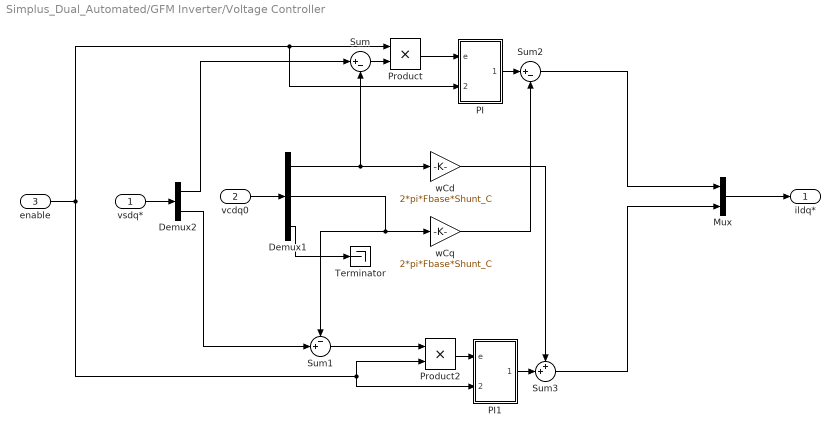
== system Simplus_Dual_Automated/GFM Inverter/Voltage Controller ==
  vsdq* : Inport
  vcdq0 : Inport  Port=2
  enable : Inport  Port=3
  Demux1 : Demux  Outputs=3
  Demux2 : Demux  Outputs=2
  Mux : Mux  Inputs=2
  PI : Subsystem
  PI1 : Subsystem
  Product : Product  RndMeth=Zero
  Product2 : Product  RndMeth=Zero
  Sum : Sum  Inputs=|+-
  Sum1 : Sum  Inputs=-+|
  Sum2 : Sum  Inputs=|+-
  Sum3 : Sum  Inputs=++|
  Terminator : Terminator
  wCd : Gain  Gain=2*pi*Fbase*Shunt_C
  wCq : Gain  Gain=2*pi*Fbase*Shunt_C
  ildq* : Outport
  wires:
  Sum2/1 -> Mux/1
  Sum3/1 -> Mux/2
  vcdq0/1 -> Demux1/1
  Mux/1 -> ildq*/1
  Demux1/3 -> Terminator/1
  vsdq*/1 -> Demux2/1
  Demux2/1 -> Sum/1
  Demux2/2 -> Sum1/2
  Product/1 -> PI/1(e)
  Sum1/1 -> Product2/1
  PI/1(Out) -> Sum2/1
  wCd/1 -> Sum3/1
  wCq/1 -> Sum2/2
  PI1/1(Out) -> Sum3/2
  Demux1/2 -> Sum1/1, wCq/1
  Demux1/1 -> wCd/1, Sum/2
  Product2/1 -> PI1/1(e)
  Sum/1 -> Product/2
  enable/1 -> Product/1, PI/2(RST), PI1/2(RST), Product2/2

== system Simplus_Dual_Automated/GFL Inverter/Current Controller Updated/PI ==
  e : Inport
  RST : Inport  Port=2
  Discrete-Time Integrator : DiscreteIntegrator  gainval=1  ExternalReset=either  SampleTime=Ts  LimitOutput=on  UpperSaturationLimit=I_SatLimit  LowerSaturationLimit=-I_SatLimit  ICPrevOutput=DiscIntNeverNeededParam  ICPrevScaledInput=DiscIntNeverNeededParam
  Ki : Gain  Gain=Id_Integral  SaturateOnIntegerOverflow=on  OutDataTypeStr=Inherit: Same as input  ParamDataTypeStr=Inherit: Same as input
  Kp : Gain  Gain=Id_Proportional  SaturateOnIntegerOverflow=on  OutDataTypeStr=Inherit: Same as input  ParamDataTypeStr=Inherit: Same as input
  Sum4 : Sum  SaturateOnIntegerOverflow=on
  Out : Outport
  tag scope: GFL_Id_Int_Out=global, GFL_Id_PI_Out=global
  wires:
  Ki/1 -> Discrete-Time Integrator/1
  Kp/1 -> Sum4/1
  e/1 -> Ki/1, Kp/1
  RST/1 -> Discrete-Time Integrator/2
  Discrete-Time Integrator/1 -> [GFL_Id_Int_Out], Sum4/2
  Sum4/1 -> [GFL_Id_PI_Out], Out/1

== system Simplus_Dual_Automated/GFL Inverter/Current Controller Updated/PI1 ==
  e : Inport
  RST : Inport  Port=2
  Discrete-Time Integrator : DiscreteIntegrator  gainval=1  ExternalReset=either  SampleTime=Ts  LimitOutput=on  UpperSaturationLimit=I_SatLimit  LowerSaturationLimit=-I_SatLimit  ICPrevOutput=DiscIntNeverNeededParam  ICPrevScaledInput=DiscIntNeverNeededParam
  Ki : Gain  Gain=Id_Integral  SaturateOnIntegerOverflow=on  OutDataTypeStr=Inherit: Same as input  ParamDataTypeStr=Inherit: Same as input
  Kp : Gain  Gain=Id_Proportional  SaturateOnIntegerOverflow=on  OutDataTypeStr=Inherit: Same as input  ParamDataTypeStr=Inherit: Same as input
  Sum4 : Sum  SaturateOnIntegerOverflow=on
  Out : Outport
  tag scope: GFL_Iq_Int_Out=global, GFL_Iq_PI_Out=global
  wires:
  Ki/1 -> Discrete-Time Integrator/1
  Kp/1 -> Sum4/1
  e/1 -> Ki/1, Kp/1
  RST/1 -> Discrete-Time Integrator/2
  Discrete-Time Integrator/1 -> [GFL_Iq_Int_Out], Sum4/2
  Sum4/1 -> [GFL_Iq_PI_Out], Out/1

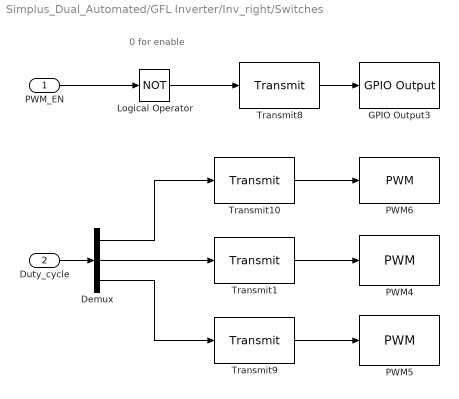
== system Simplus_Dual_Automated/GFL Inverter/Inv_right/Switches ==
  note: 0 for enable
  PWM_EN : Inport
  Duty_cycle : Inport  Port=2
  Demux : Demux  Outputs=3
  GPIO Output3 : rtpi/GPIO Output  finger_print=115482637925  blk_num=1  gpio_num=1  gpio1=24  od1=off  gpio2=0  od2=off  gpio3=0  od3=off  gpio4=0  od4=off  gpio5=0  od5=off  gpio6=0  od6=off  gpio7=0  od7=off  gpio8=0  od8=off  gpio9=0  od9=off  gpio10=0  od10=off  gpio11=0  od11=off  gpio12=0  od12=off  gpio13=0  od13=off  gpio14=0  od14=off  gpio15=0  od15=off  gpio16=0  od16=off  dir=1
      settings: SourceProductName=Simplus Real-Time
  Logical Operator : Logic  Operator=NOT  AllPortsSameDT=off  OutDataTypeStr=boolean
  PWM4 : rtpi/PWM  finger_print=115482637925  blk_num=1  pwmx=2  sync=on  mode=Normal  input=Duty Cycle  data_type=float  trigger_a=Zero  trigger_b=Zero  clock=1  tdead=2  period=10000  duty=0.5  phase=0.0
      settings: SourceProductName=Simplus Real-Time
  PWM5 : rtpi/PWM  finger_print=115482637925  blk_num=2  pwmx=3  sync=on  mode=Normal  input=Duty Cycle  data_type=float  trigger_a=Zero  trigger_b=Zero  clock=1  tdead=2  period=10000  duty=0.5  phase=0.0
      settings: SourceProductName=Simplus Real-Time
  PWM6 : rtpi/PWM  finger_print=115482637925  blk_num=3  pwmx=1  sync=on  mode=Normal  input=Duty Cycle  data_type=float  trigger_a=Zero  trigger_b=Zero  clock=1  tdead=2  period=10000  duty=0.5  phase=0.0
      settings: SourceProductName=Simplus Real-Time
  Transmit1 : rtpi/Transmit  Priority=10  finger_print=115482637925  blk_num=1  data_type=4  conv_type=single
      settings: SourceProductName=Simplus Real-Time
  Transmit10 : rtpi/Transmit  Priority=10  finger_print=115482637925  blk_num=2  data_type=4  conv_type=single
      settings: SourceProductName=Simplus Real-Time
  Transmit8 : rtpi/Transmit  finger_print=115482637925  blk_num=3  data_type=2  conv_type=uint16
      settings: SourceProductName=Simplus Real-Time
  Transmit9 : rtpi/Transmit  Priority=10  finger_print=115482637925  blk_num=4  data_type=4  conv_type=single
      settings: SourceProductName=Simplus Real-Time
  wires:
  Duty_cycle/1 -> Demux/1
  PWM_EN/1 -> Logical Operator/1
  Demux/3 -> Transmit9/1
  Demux/1 -> Transmit10/1
  Demux/2 -> Transmit1/1
  Transmit9/1 -> PWM5/1
  Transmit1/1 -> PWM4/1
  Transmit10/1 -> PWM6/1
  Transmit8/1 -> GPIO Output3/1
  Logical Operator/1 -> Transmit8/1

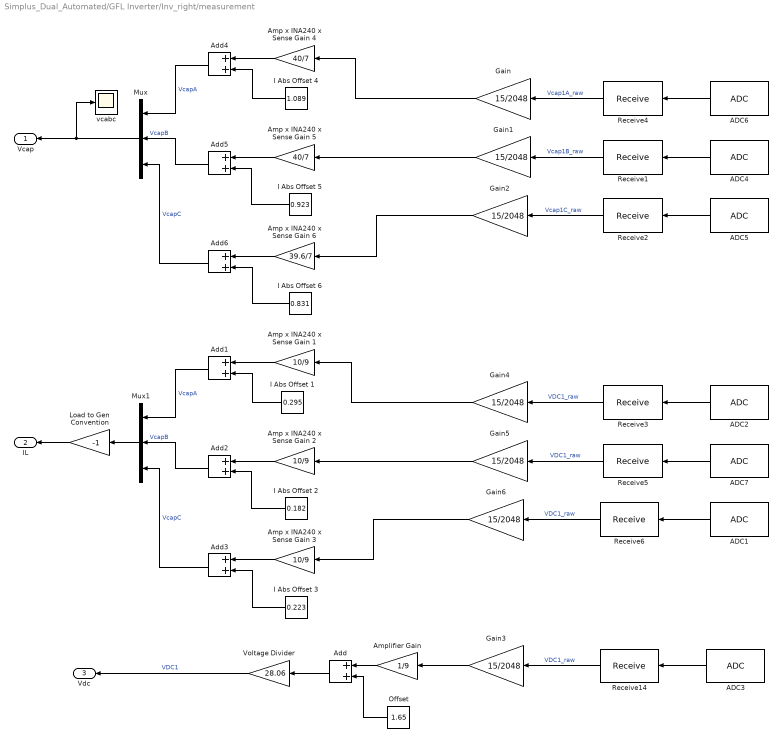
== system Simplus_Dual_Automated/GFL Inverter/Inv_right/measurement ==
  ADC1 : rtpi/ADC  finger_print=115482637925  blk_num=1  adcx=A  prior=1  pin=A1  trigger=PWM1A  data_type=int16  gain=1  rsrc=100  offset=AC  protect=Enabled  max=1500  min=-1500
      settings: SourceProductName=Simplus Real-Time
  ADC2 : rtpi/ADC  finger_print=115482637925  blk_num=2  adcx=A  prior=2  pin=A2  trigger=PWM1A  data_type=int16  gain=1  rsrc=100  offset=AC  protect=Enabled  max=1500  min=-1500
      settings: SourceProductName=Simplus Real-Time
  ADC3 : rtpi/ADC  finger_print=115482637925  blk_num=3  adcx=A  prior=4  pin=A4  trigger=PWM1A  data_type=int16  gain=1  rsrc=100  offset=AC  protect=Enabled  max=1500  min=-2048
      settings: SourceProductName=Simplus Real-Time
  ADC4 : rtpi/ADC  finger_print=115482637925  blk_num=4  adcx=B  prior=2  pin=B3  trigger=PWM1A  data_type=int16  gain=1  rsrc=100  offset=AC  protect=Enabled  max=1500  min=-1500
      settings: SourceProductName=Simplus Real-Time
  ADC5 : rtpi/ADC  finger_print=115482637925  blk_num=5  adcx=B  prior=3  pin=B4  trigger=PWM1A  data_type=int16  gain=1  rsrc=100  offset=AC  protect=Enabled  max=1500  min=-1500
      settings: SourceProductName=Simplus Real-Time
  ADC6 : rtpi/ADC  finger_print=115482637925  blk_num=6  adcx=B  prior=1  pin=B2  trigger=PWM1A  data_type=int16  gain=1  rsrc=100  offset=AC  protect=Enabled  max=1500  min=-1500
      settings: SourceProductName=Simplus Real-Time
  ADC7 : rtpi/ADC  finger_print=115482637925  blk_num=7  adcx=A  prior=3  pin=A3  trigger=PWM1A  data_type=int16  gain=1  rsrc=100  offset=AC  protect=Enabled  max=1500  min=-1500
      settings: SourceProductName=Simplus Real-Time
  Add{,1..6} (7 alike) : Sum
  Amp x INA240 x Sense Gain 1 : Gain  Gain=10/9
  Amp x INA240 x Sense Gain 2 : Gain  Gain=10/9
  Amp x INA240 x Sense Gain 3 : Gain  Gain=10/9
  Amp x INA240 x Sense Gain 4 : Gain  Gain=40/7
  Amp x INA240 x Sense Gain 5 : Gain  Gain=40/7
  Amp x INA240 x Sense Gain 6 : Gain  Gain=39.6/7
  Amplifier Gain : Gain  Gain=1/9
  Gain{,1..6} (7 alike) : Gain  Gain=15/2048
  I Abs Offset 1 : Constant  Value=0.295
  I Abs Offset 2 : Constant  Value=0.182
  I Abs Offset 3 : Constant  Value=0.223
  I Abs Offset 4 : Constant  Value=1.089
  I Abs Offset 5 : Constant  Value=0.923
  I Abs Offset 6 : Constant  Value=0.831
  Load to Gen Convention : Gain  Gain=-1
  Mux : Mux  Inputs=3
  Mux1 : Mux  Inputs=3
  Offset : Constant  Value=1.65
  Receive1 : rtpi/Receive  Priority=12  finger_print=115482637925  blk_num=1  data_type=2
      settings: SourceProductName=Simplus Real-Time
  Receive14 : rtpi/Receive  Priority=12  finger_print=115482637925  blk_num=2  data_type=2
      settings: SourceProductName=Simplus Real-Time
  Receive2 : rtpi/Receive  Priority=12  finger_print=115482637925  blk_num=3  data_type=2
      settings: SourceProductName=Simplus Real-Time
  Receive3 : rtpi/Receive  Priority=12  finger_print=115482637925  blk_num=4  data_type=2
      settings: SourceProductName=Simplus Real-Time
  Receive4 : rtpi/Receive  Priority=12  finger_print=115482637925  blk_num=5  data_type=2
      settings: SourceProductName=Simplus Real-Time
  Receive5 : rtpi/Receive  Priority=12  finger_print=115482637925  blk_num=6  data_type=2
      settings: SourceProductName=Simplus Real-Time
  Receive6 : rtpi/Receive  Priority=12  finger_print=115482637925  blk_num=7  data_type=2
      settings: SourceProductName=Simplus Real-Time
  Voltage Divider : Gain  Gain=28.06
  vcabc : Scope
  Vcap : Outport
  IL : Outport  Port=2
  Vdc : Outport  Port=3
  wires:
  ADC6/1 -> Receive4/1
  Receive4/1 -> Gain/1  "Vcap1A_raw"
  Amp x INA240 x Sense Gain 6/1 -> Add6/1
  I Abs Offset 6/1 -> Add6/2
  I Abs Offset 4/1 -> Add4/2
  Amp x INA240 x Sense Gain 4/1 -> Add4/1
  ADC5/1 -> Receive2/1
  Amp x INA240 x Sense Gain 5/1 -> Add5/1
  Receive1/1 -> Gain1/1  "Vcap1B_raw"
  I Abs Offset 5/1 -> Add5/2
  Receive2/1 -> Gain2/1  "Vcap1C_raw"
  ADC4/1 -> Receive1/1
  Amp x INA240 x Sense Gain 3/1 -> Add3/1
  Amp x INA240 x Sense Gain 1/1 -> Add1/1
  I Abs Offset 1/1 -> Add1/2
  Amp x INA240 x Sense Gain 2/1 -> Add2/1
  I Abs Offset 2/1 -> Add2/2
  I Abs Offset 3/1 -> Add3/2
  Receive14/1 -> Gain3/1  "VDC1_raw"
  ADC3/1 -> Receive14/1
  Add/1 -> Voltage Divider/1
  Voltage Divider/1 -> Vdc/1  "VDC1"
  Amplifier Gain/1 -> Add/1
  Offset/1 -> Add/2
  Gain/1 -> Amp x INA240 x Sense Gain 4/1
  Gain1/1 -> Amp x INA240 x Sense Gain 5/1
  Gain2/1 -> Amp x INA240 x Sense Gain 6/1
  Gain3/1 -> Amplifier Gain/1
  Add4/1 -> Mux/1  "VcapA"
  Add5/1 -> Mux/2  "VcapB"
  Add6/1 -> Mux/3  "VcapC"
  Gain4/1 -> Amp x INA240 x Sense Gain 1/1
  Gain5/1 -> Amp x INA240 x Sense Gain 2/1
  Gain6/1 -> Amp x INA240 x Sense Gain 3/1
  Add3/1 -> Mux1/3  "VcapC"
  Mux1/1 -> Load to Gen Convention/1
  Add1/1 -> Mux1/1  "VcapA"
  Add2/1 -> Mux1/2  "VcapB"
  Receive3/1 -> Gain4/1  "VDC1_raw"
  ADC2/1 -> Receive3/1
  Receive5/1 -> Gain5/1  "VDC1_raw"
  ADC7/1 -> Receive5/1
  Receive6/1 -> Gain6/1  "VDC1_raw"
  ADC1/1 -> Receive6/1
  Load to Gen Convention/1 -> IL/1
  Mux/1 -> vcabc/1, Vcap/1

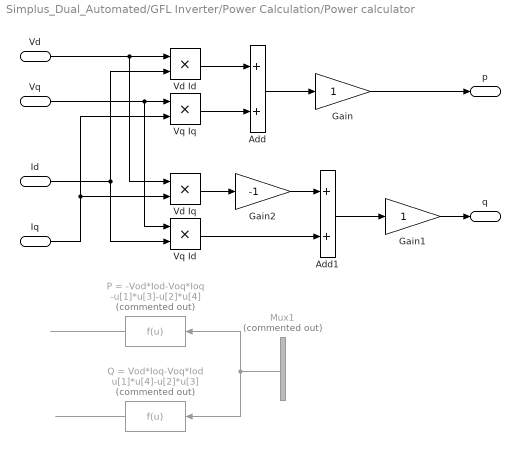
== system Simplus_Dual_Automated/GFL Inverter/Power Calculation/Power calculator ==
  Vd : Inport
  Vq : Inport  Port=2
  Id : Inport  Port=3
  Iq : Inport  Port=4
  Add : Sum
  Add1 : Sum
  Gain : Gain
  Gain1 : Gain
  Gain2 : Gain  Gain=-1
  Mux1 : Mux  Commented=on
  P = -Vod*Iod-Voq*Ioq : Fcn  Commented=on  Expr=-u[1]*u[3]-u[2]*u[4]
  Q = Vod*Ioq-Voq*Iod : Fcn  Commented=on  Expr=u[1]*u[4]-u[2]*u[3]
  Vd Id : Product
  Vd Iq : Product
  Vq Id : Product
  Vq Iq : Product
  p : Outport
  q : Outport  Port=2
  wires:
  Q = Vod*Ioq-Voq*Iod/1 -> ?
  P = -Vod*Iod-Voq*Ioq/1 -> ?
  Mux1/1 -> Q = Vod*Ioq-Voq*Iod/1, P = -Vod*Iod-Voq*Ioq/1
  Gain/1 -> p/1
  Add/1 -> Gain/1
  Add1/1 -> Gain1/1
  Gain1/1 -> q/1
  Vd Id/1 -> Add/1
  Vq Iq/1 -> Add/2
  Vq Id/1 -> Add1/2
  Vd Iq/1 -> Gain2/1
  Vd/1 -> Vd Iq/1, Vd Id/1
  Id/1 -> Vd Id/2, Vq Id/2
  Vq/1 -> Vq Id/1, Vq Iq/1
  Iq/1 -> Vd Iq/2, Vq Iq/2
  Gain2/1 -> Add1/1

== system Simplus_Dual_Automated/GFM Inverter/Current Controller Updated1/PI ==
  e : Inport
  RST : Inport  Port=2
  Discrete-Time Integrator : DiscreteIntegrator  gainval=1  ExternalReset=either  SampleTime=Ts  LimitOutput=on  UpperSaturationLimit=I_IntSat  LowerSaturationLimit=-I_IntSat  ICPrevOutput=DiscIntNeverNeededParam  ICPrevScaledInput=DiscIntNeverNeededParam
  Ki : Gain  Gain=Id_Integral  SaturateOnIntegerOverflow=on  OutDataTypeStr=Inherit: Same as input  ParamDataTypeStr=Inherit: Same as input
  Kp : Gain  Gain=Id_Proportional  SaturateOnIntegerOverflow=on  OutDataTypeStr=Inherit: Same as input  ParamDataTypeStr=Inherit: Same as input
  Sum4 : Sum  SaturateOnIntegerOverflow=on
  Out : Outport
  tag scope: GFM_Id_Int_Out=global, GFM_Id_PI_Out=global
  wires:
  Ki/1 -> Discrete-Time Integrator/1
  Kp/1 -> Sum4/1
  e/1 -> Ki/1, Kp/1
  RST/1 -> Discrete-Time Integrator/2
  Discrete-Time Integrator/1 -> [GFM_Id_Int_Out], Sum4/2
  Sum4/1 -> [GFM_Id_PI_Out], Out/1

== system Simplus_Dual_Automated/GFM Inverter/Current Controller Updated1/PI1 ==
  e : Inport
  RST : Inport  Port=2
  Discrete-Time Integrator : DiscreteIntegrator  gainval=1  ExternalReset=either  SampleTime=Ts  LimitOutput=on  UpperSaturationLimit=I_IntSat  LowerSaturationLimit=-I_IntSat  ICPrevOutput=DiscIntNeverNeededParam  ICPrevScaledInput=DiscIntNeverNeededParam
  Ki : Gain  Gain=Id_Integral  SaturateOnIntegerOverflow=on  OutDataTypeStr=Inherit: Same as input  ParamDataTypeStr=Inherit: Same as input
  Kp : Gain  Gain=Id_Proportional  SaturateOnIntegerOverflow=on  OutDataTypeStr=Inherit: Same as input  ParamDataTypeStr=Inherit: Same as input
  Sum4 : Sum  SaturateOnIntegerOverflow=on
  Out : Outport
  tag scope: GFM_Iq_Int_Out=global, GFM_Iq_PI_Out=global
  wires:
  Ki/1 -> Discrete-Time Integrator/1
  Kp/1 -> Sum4/1
  e/1 -> Ki/1, Kp/1
  RST/1 -> Discrete-Time Integrator/2
  Discrete-Time Integrator/1 -> [GFM_Iq_Int_Out], Sum4/2
  Sum4/1 -> [GFM_Iq_PI_Out], Out/1

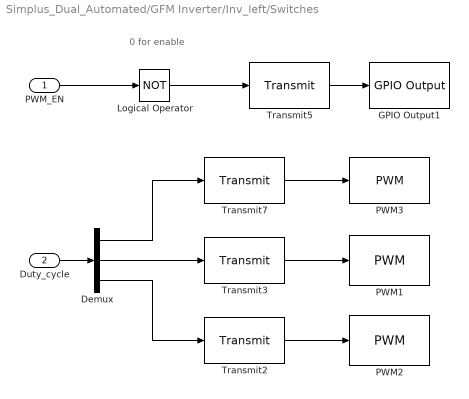
== system Simplus_Dual_Automated/GFM Inverter/Inv_left/Switches ==
  note: 0 for enable
  PWM_EN : Inport
  Duty_cycle : Inport  Port=2
  Demux : Demux  Outputs=3
  GPIO Output1 : rtpi/GPIO Output  finger_print=115482637925  blk_num=2  gpio_num=1  gpio1=18  od1=off  gpio2=0  od2=off  gpio3=0  od3=off  gpio4=0  od4=off  gpio5=0  od5=off  gpio6=0  od6=off  gpio7=0  od7=off  gpio8=0  od8=off  gpio9=0  od9=off  gpio10=0  od10=off  gpio11=0  od11=off  gpio12=0  od12=off  gpio13=0  od13=off  gpio14=0  od14=off  gpio15=0  od15=off  gpio16=0  od16=off  dir=1
      settings: SourceProductName=Simplus Real-Time
  Logical Operator : Logic  Operator=NOT  AllPortsSameDT=off  OutDataTypeStr=boolean
  PWM1 : rtpi/PWM  finger_print=115482637925  blk_num=4  pwmx=5  sync=on  mode=Normal  input=Duty Cycle  data_type=float  trigger_a=Zero  trigger_b=Zero  clock=1  tdead=2  period=10000  duty=0.5  phase=0.0
      settings: SourceProductName=Simplus Real-Time
  PWM2 : rtpi/PWM  finger_print=115482637925  blk_num=5  pwmx=6  sync=on  mode=Normal  input=Duty Cycle  data_type=float  trigger_a=Zero  trigger_b=Zero  clock=1  tdead=2  period=10000  duty=0.5  phase=0.0
      settings: SourceProductName=Simplus Real-Time
  PWM3 : rtpi/PWM  finger_print=115482637925  blk_num=6  pwmx=4  sync=on  mode=Normal  input=Duty Cycle  data_type=float  trigger_a=Zero  trigger_b=Zero  clock=1  tdead=2  period=10000  duty=0.5  phase=0.0
      settings: SourceProductName=Simplus Real-Time
  Transmit2 : rtpi/Transmit  Priority=10  finger_print=115482637925  blk_num=5  data_type=4  conv_type=single
      settings: SourceProductName=Simplus Real-Time
  Transmit3 : rtpi/Transmit  Priority=10  finger_print=115482637925  blk_num=6  data_type=4  conv_type=single
      settings: SourceProductName=Simplus Real-Time
  Transmit5 : rtpi/Transmit  finger_print=115482637925  blk_num=7  data_type=2  conv_type=uint16
      settings: SourceProductName=Simplus Real-Time
  Transmit7 : rtpi/Transmit  Priority=10  finger_print=115482637925  blk_num=8  data_type=4  conv_type=single
      settings: SourceProductName=Simplus Real-Time
  wires:
  Transmit2/1 -> PWM2/1
  Transmit3/1 -> PWM1/1
  Transmit7/1 -> PWM3/1
  Duty_cycle/1 -> Demux/1
  Demux/2 -> Transmit3/1
  Demux/1 -> Transmit7/1
  Demux/3 -> Transmit2/1
  Transmit5/1 -> GPIO Output1/1
  Logical Operator/1 -> Transmit5/1
  PWM_EN/1 -> Logical Operator/1
